simulink model "forwardInverse"  (R2022b)
settings: Solver=VariableStepAuto  StartTime=0.0  StopTime=10.0  RelTol=1e-3
settings Model: Creator=sathwik  LastModifiedBy=sathwik

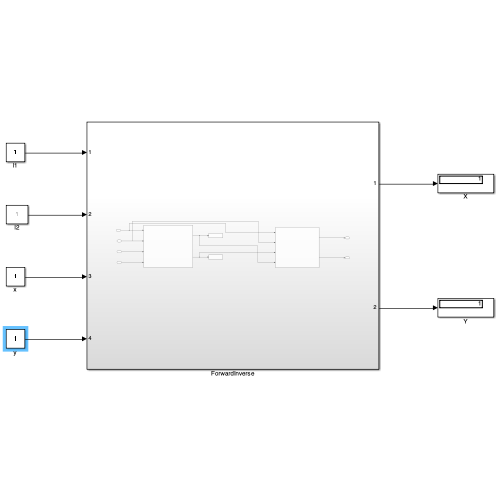
[thumbnail: Simulink's stored preview of the top-level diagram]
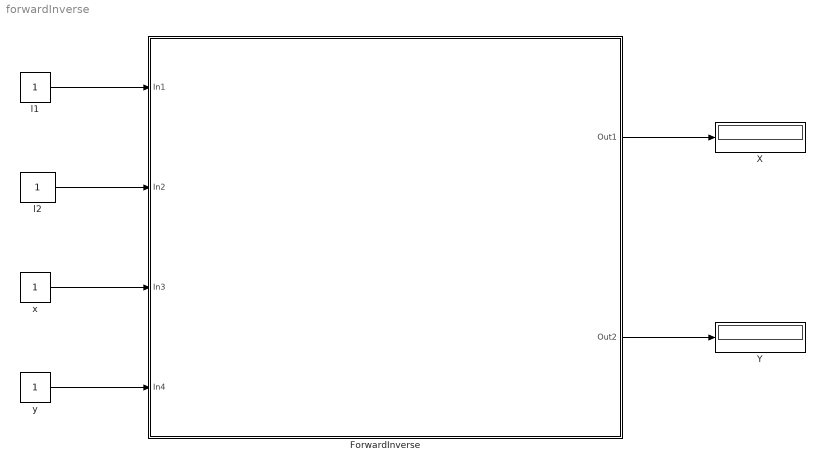
== system forwardInverse ==
  ForwardInverse : Subsystem
  X : Display
  Y : Display
  l1 : Constant
  l2 : Constant
  x : Constant
  y : Constant
  wires:
  l1/1 -> ForwardInverse/1(In1)
  l2/1 -> ForwardInverse/2(In2)
  x/1 -> ForwardInverse/3(In3)
  y/1 -> ForwardInverse/4(In4)
  ForwardInverse/1(Out1) -> X/1
  ForwardInverse/2(Out2) -> Y/1

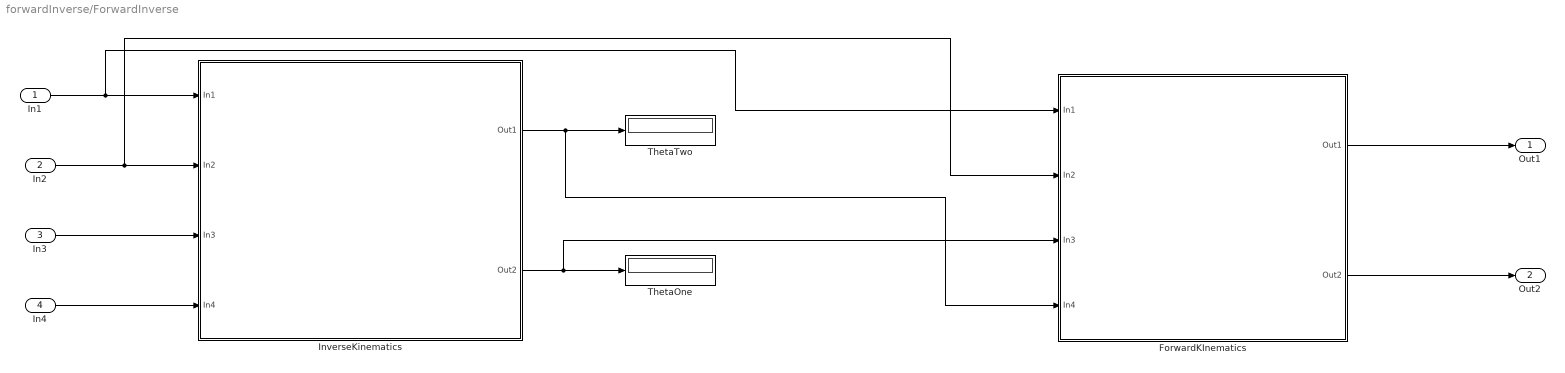
== system forwardInverse/ForwardInverse ==
  In1 : Inport
  In2 : Inport  Port=2
  In3 : Inport  Port=3
  In4 : Inport  Port=4
  ForwardKInematics : Subsystem
  InverseKinematics : Subsystem
  ThetaOne : Display
  ThetaTwo : Display
  Out1 : Outport
  Out2 : Outport  Port=2
  wires:
  In4/1 -> InverseKinematics/4(In4)
  In3/1 -> InverseKinematics/3(In3)
  ForwardKInematics/1(Out1) -> Out1/1
  In1/1 -> ForwardKInematics/1(In1), InverseKinematics/1(In1)
  ForwardKInematics/2(Out2) -> Out2/1
  In2/1 -> ForwardKInematics/2(In2), InverseKinematics/2(In2)
  InverseKinematics/2(Out2) -> ForwardKInematics/3(In3), ThetaOne/1
  InverseKinematics/1(Out1) -> ForwardKInematics/4(In4), ThetaTwo/1

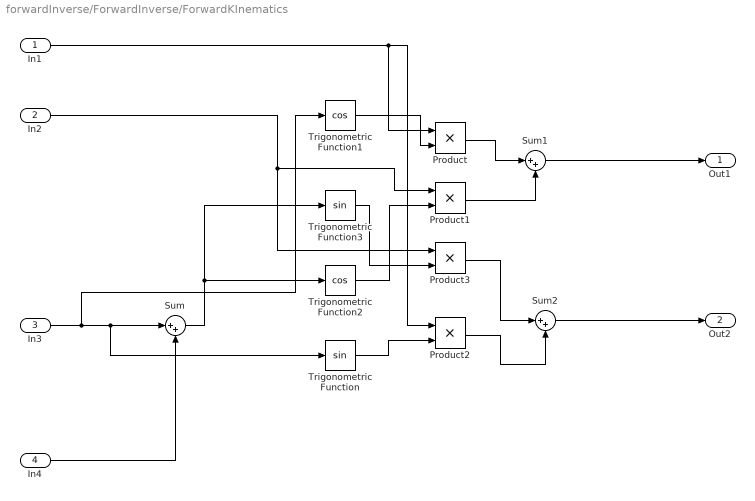
== system forwardInverse/ForwardInverse/ForwardKInematics ==
  In1 : Inport
  In2 : Inport  Port=2
  In3 : Inport  Port=3
  In4 : Inport  Port=4
  Product{,1..3} (4 alike) : Product
  Sum : Sum  Inputs=|++
  Sum1 : Sum  Inputs=|++
  Sum2 : Sum  Inputs=|++
  Trigonometric Function : Trigonometry
  Trigonometric Function1 : Trigonometry  Operator=cos
  Trigonometric Function2 : Trigonometry  Operator=cos
  Trigonometric Function3 : Trigonometry
  Out1 : Outport
  Out2 : Outport  Port=2
  wires:
  Sum2/1 -> Out2/1
  In4/1 -> Sum/2
  Sum1/1 -> Out1/1
  Product3/1 -> Sum2/1
  In1/1 -> Product2/1, Product/1
  Product/1 -> Sum1/1
  Product1/1 -> Sum1/2
  Trigonometric Function1/1 -> Product/2
  Sum/1 -> Trigonometric Function3/1, Trigonometric Function2/1
  Product2/1 -> Sum2/2
  In2/1 -> Product3/1, Product1/1
  Trigonometric Function2/1 -> Product1/2
  Trigonometric Function3/1 -> Product3/2
  In3/1 -> Trigonometric Function1/1, Trigonometric Function/1, Sum/1
  Trigonometric Function/1 -> Product2/2

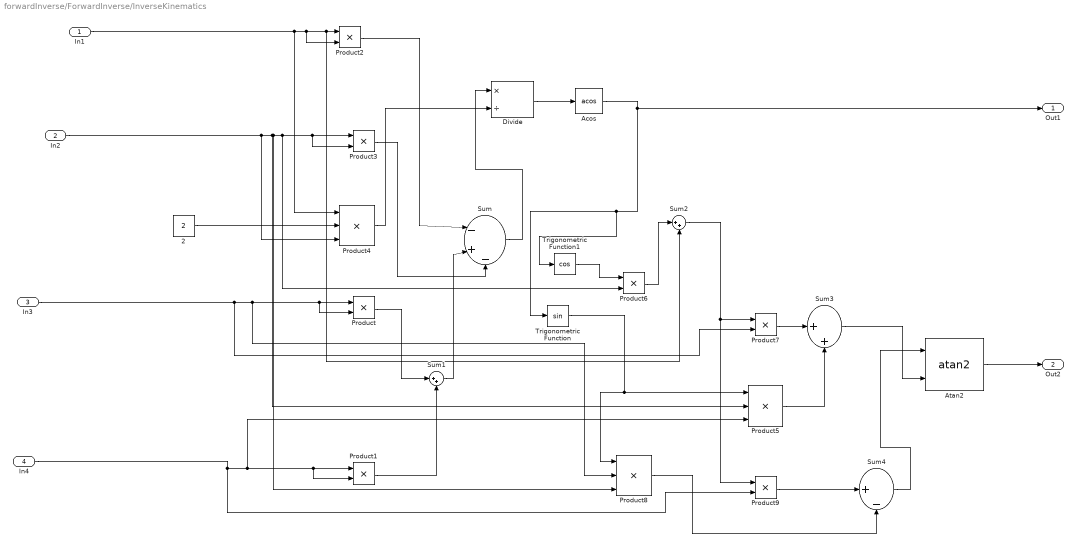
== system forwardInverse/ForwardInverse/InverseKinematics ==
  In1 : Inport
  In2 : Inport  Port=2
  In3 : Inport  Port=3
  In4 : Inport  Port=4
  2 : Constant  Value=2
  Acos : Trigonometry  Operator=acos
  Atan2 : Trigonometry  Operator=atan2
  Divide : Product  Inputs=*/
  Product{,1..3,6..7,9} (7 alike) : Product
  Product4 : Product  Inputs=3
  Product5 : Product  Inputs=3
  Product8 : Product  Inputs=3
  Sum : Sum  Inputs=|-+-
  Sum1 : Sum  Inputs=|++
  Sum2 : Sum  Inputs=|++
  Sum3 : Sum  Inputs=|++
  Sum4 : Sum  Inputs=|+-
  Trigonometric Function : Trigonometry
  Trigonometric Function1 : Trigonometry  Operator=cos
  Out1 : Outport
  Out2 : Outport  Port=2
  wires:
  Product8/1 -> Sum4/2
  Product4/1 -> Divide/2
  Product7/1 -> Sum3/1
  Atan2/1 -> Out2/1
  Sum/1 -> Divide/1
  In2/1 -> Product8/3, Product6/2, Product3/2, Product3/1, Product5/2, Product4/3
  Product5/1 -> Sum3/2
  Product2/1 -> Sum/1
  Product3/1 -> Sum/3
  Product6/1 -> Sum2/1
  In3/1 -> Product7/2, Product8/2, Product/2, Product/1
  In4/1 -> Product9/2, Product5/3, Product1/2, Product1/1
  Product/1 -> Sum1/1
  2/1 -> Product4/2
  Acos/1 -> Out1/1, Trigonometric Function1/1, Trigonometric Function/1
  Sum4/1 -> Atan2/1
  In1/1 -> Sum2/2, Product2/1, Product2/2, Product4/1
  Divide/1 -> Acos/1
  Sum1/1 -> Sum/2
  Sum2/1 -> Product9/1, Product7/1
  Sum3/1 -> Atan2/2
  Trigonometric Function1/1 -> Product6/1
  Product1/1 -> Sum1/2
  Product9/1 -> Sum4/1
  Trigonometric Function/1 -> Product8/1, Product5/1
